simulink model "SELECTOR"  (R2021a)
settings: Solver=VariableStepAuto  StartTime=0.0  StopTime=inf  RelTol=1e-3
libraries: instrumentseriallib x2
settings Model: Creator=ashle  LastModifiedBy=mgn16
settings SolverCC: AlgebraicLoopSolver=TrustRegion
settings DebuggingCC: SFMachineParentedDataDiag=warning
settings SFSimCC: CustomCodeUndefinedFunction=UseInterfaceOnly

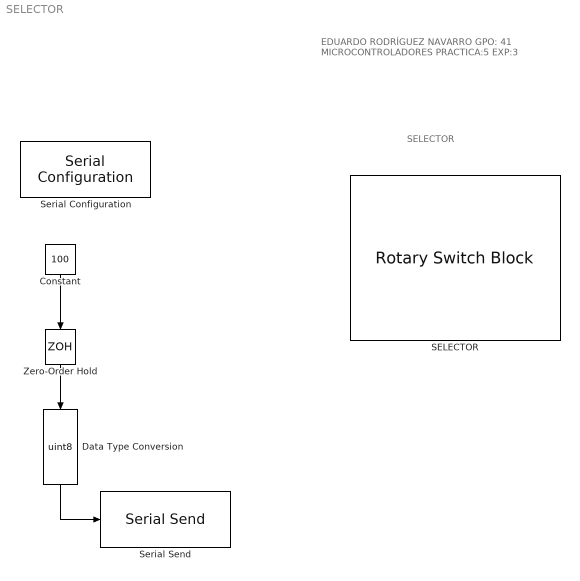
== system SELECTOR ==
  note: EDUARDO RODRÍGUEZ NAVARRO
      | GPO: 41
      | MICROCONTROLADORES
      | PRACTICA:5 EXP:3
  note: SELECTOR
  "Constant " : Constant  Value=100
  Data Type Conversion : DataTypeConversion  OutDataTypeStr=uint8
  "SELECTOR " : RotarySwitchBlock
      settings: Values={{'0 %', '10 %', '20 %', '30 %', '40 %', '50 %', '60 %', '70 %', '80 %', '90 %', '100 %', 'Rojo', 'Verde', 'Azul'}, [1 10 20 30 40 50 60 70 80 90 100 114 103 98]}
  "Serial Configuration " : instrumentseriallib/Serial Configuration  Priority=-200000  Port=COM7  ComPort=COM7  BaudRate=9600  DataBits=8  Parity=none  StopBits=1  ByteOrder=little-endian  FlowControl=none  Timeout=10  SimulateUsing=Interpreted execution  BlockInModel=on
  "Serial Send " : instrumentseriallib/Serial Send  Port=<Select a port...>  ComPort=<Select a port...>  Header=[]  Terminator=<none>  CustomTerminator=[]  EnableBlockingMode=on  SimulateUsing=Interpreted execution  BlockInModel=on
  "Zero-Order Hold " : ZeroOrderHold  SampleTime=0.5
  wires:
  Data Type Conversion/1 -> "Serial Send "/1
  "Constant "/1 -> "Zero-Order Hold "/1
  "Zero-Order Hold "/1 -> Data Type Conversion/1
